simulink model "test_direct"  (R2024a)
settings: Solver=VariableStepAuto  StartTime=0.0  StopTime=40  RelTol=1e-3
libraries: neural x733, simulink x4
(part 12 of 35)

== system test_direct/Function Fitting Neural Network1/Layer 4/Delays 1 ==
  "p{4}" : Inport  PortDimensions=20
      mask Display: e = 0.06;c1 = [120 230 180]/255;c2 = ([120 230 180]+0)/(256+128);c3 = ([120 230 180]+128)/(256+128);patch([0 1 1 0],[0 0 1 1],c1);patch([0 1 1 1-e 1-e 0+e],[0 0 1 1-e 0+e 0+e],c2);patch([0 0 1 1-e 0+e 0+e],[0 1 1 1-e 1-e 0+e],c3);plot([0 1 1 0 0],[0 0 1 1 0]);
  mux : Mux  Inputs=1
      mask Display: e = 0.06;c1 = [120 150 230]/255;c2 = ([120 150 230]+0)/383;c3 = ([120 150 230]+128)/383;patch([0 1 1 0],[0 0 1 1],c1);patch([0 1 1 1-e 1-e 0+e],[0 0 1 1-e 0+e 0+e],c2);patch([0 0 1 1-e 0+e 0+e],[0 1 1 1-e 1-e 0+e],c3);plot([0 1 1 0 0],[0 0 1 1 0]);disp('Mux')
  "pd{4,3}" : Outport
      mask Display: e = 0.06;c1 = [120 230 180]/255;c2 = ([120 230 180]+0)/(256+128);c3 = ([120 230 180]+128)/(256+128);patch([0 1 1 0],[0 0 1 1],c1);patch([0 1 1 1-e 1-e 0+e],[0 0 1 1-e 0+e 0+e],c2);patch([0 0 1 1-e 0+e 0+e],[0 1 1 1-e 1-e 0+e],c3);plot([0 1 1 0 0],[0 0 1 1 0]);
  wires:
  "p{4}"/1 -> mux/1
  mux/1 -> "pd{4,3}"/1

== system test_direct/Function Fitting Neural Network1/Layer 4/LW{4,3} ==
  "ad{4,3}" : Inport  PortDimensions=20
      mask Display: e = 0.06;c1 = [120 230 180]/255;c2 = ([120 230 180]+0)/(256+128);c3 = ([120 230 180]+128)/(256+128);patch([0 1 1 0],[0 0 1 1],c1);patch([0 1 1 1-e 1-e 0+e],[0 0 1 1-e 0+e 0+e],c2);patch([0 0 1 1-e 0+e 0+e],[0 1 1 1-e 1-e 0+e],c3);plot([0 1 1 0 0],[0 0 1 1 0]);
  "IW{4,3}(1,:)'" : Constant  Value=[-0.5538978955091093947515901163569651544094085693359375;0.485168151202809372346536065379041247069835662841796875;-0.5241552760058165727485857132705859839916229248046875;0.393694130681727594289753824341460131108760833740234375;-0.226868820201836685068741417126148007810115814208984375;-0.57887128109770780159948344589793123304843902587890625;-0.0783114975214572461847950535229756496846675872802734375;-0.045766236741898003170803121975040994584560394287109375;0.399668940356752655507222016240120865404605865478515625;0.1856571666806976772523540830661659128963947296142578125;0.10022603350572274749641366042851586826145648956298828125;-0.534264069916555950356951143476180732250213623046875;-0.32018358640142363658043223040294833481311798095703125;0.0185677915168835395987034786458025337196886539459228515625;0.191883392055136547948990255463286302983760833740234375;-0.2105355645822364618613420361725729890167713165283203125;-0.5841688118866372736448511204798705875873565673828125;-0.1594929997566735535574622417698265053331851959228515625;-0.335012858362053245198097783941193483769893646240234375;0.115969582185506958627030371644650585949420928955078125]
      mask Display: e = 0.06;c1 = [120 150 230]/255;c2 = ([120 150 230]+0)/383;c3 = ([120 150 230]+128)/383;patch([0 1 1 0],[0 0 1 1],c1);patch([0 1 1 1-e 1-e 0+e],[0 0 1 1-e 0+e 0+e],c2);patch([0 0 1 1-e 0+e 0+e],[0 1 1 1-e 1-e 0+e],c3);plot([0 1 1 0 0],[0 0 1 1 0]);disp('weights');
  "IW{4,3}(10,:)'" : Constant  Value=[-0.11432279213753747393322868219911470077931880950927734375;-0.482351266656278365729804136208258569240570068359375;-0.401522130496478724115405611883033998310565948486328125;0.240701254689964783128885983387590385973453521728515625;0.463959354447395833087597338817431591451168060302734375;-0.0857875597282283519628975909654400311410427093505859375;-0.464149306377789672151124023002921603620052337646484375;-0.08157369651331071447319942535614245571196079254150390625;-0.0184508443188259076139789982562433579005300998687744140625;0.10195442949925893894036477149711572565138339996337890625;-0.44268411642938565453420096673653461039066314697265625;0.07689143542623187721485322754233493469655513763427734375;-0.5351185554038793146247598997433669865131378173828125;-0.55882335224635160120243426717934198677539825439453125;-0.3511500841433623509857397948508150875568389892578125;0.053339980043120759078956183429909287951886653900146484375;0.250608480405577427330143791550653986632823944091796875;-0.48472883013925793793674756670952774584293365478515625;-0.4930568315285324132446476141922175884246826171875;-0.260318494558593072074614838129491545259952545166015625]
      mask Display: e = 0.06;c1 = [120 150 230]/255;c2 = ([120 150 230]+0)/383;c3 = ([120 150 230]+128)/383;patch([0 1 1 0],[0 0 1 1],c1);patch([0 1 1 1-e 1-e 0+e],[0 0 1 1-e 0+e 0+e],c2);patch([0 0 1 1-e 0+e 0+e],[0 1 1 1-e 1-e 0+e],c3);plot([0 1 1 0 0],[0 0 1 1 0]);disp('weights');
  "IW{4,3}(2,:)'" : Constant  Value=[0.0127625592697413470233414045651443302631378173828125;-0.2491011110049460575144308904782519675791263580322265625;0.274529221095729691892728396851452998816967010498046875;0.0204354876268000480721287459573431988246738910675048828125;0.1585695336445297753957817121772677637636661529541015625;-0.433717579824423993262172416507382877171039581298828125;0.256549476269036180742233455021050758659839630126953125;-0.59634213250017176211059677370940335094928741455078125;0.467939192879395393642738554262905381619930267333984375;-0.5351803245451469681626122110174037516117095947265625;0.306031635985715144698815493029542267322540283203125;0.60240914911445175849991073846467770636081695556640625;-0.272057168040332530978275826782919466495513916015625;-0.11290972902060793237044578063432709313929080963134765625;-0.272119262681239593160142931083100847899913787841796875;0.33969783556142285618761889054439961910247802734375;-0.336592646572185183462266877540969289839267730712890625;-0.0674673853582745675083742753486149013042449951171875;0.02810640498377771356874887942467466928064823150634765625;-0.56221562973156402609475890130852349102497100830078125]
      mask Display: e = 0.06;c1 = [120 150 230]/255;c2 = ([120 150 230]+0)/383;c3 = ([120 150 230]+128)/383;patch([0 1 1 0],[0 0 1 1],c1);patch([0 1 1 1-e 1-e 0+e],[0 0 1 1-e 0+e 0+e],c2);patch([0 0 1 1-e 0+e 0+e],[0 1 1 1-e 1-e 0+e],c3);plot([0 1 1 0 0],[0 0 1 1 0]);disp('weights');
  "IW{4,3}(3,:)'" : Constant  Value=[0.2188595104604072194565134168442455120384693145751953125;-0.61082191094920623708475204693968407809734344482421875;-0.13949203191923309486099924470181576907634735107421875;0.088990754412494210701112251626909710466861724853515625;-0.2483977615196539534547781613582628779113292694091796875;0.64019161482434838728039494526456110179424285888671875;0.055384886144940685681614667146277497522532939910888671875;0.134629674044515368347418871053378097712993621826171875;-0.334046415075910541059300840061041526496410369873046875;-0.31450471701658344603202976941247470676898956298828125;0.468475534970048623772953533261897973716259002685546875;-0.225258262897470029617608133776229806244373321533203125;-0.79555667711204380854184137206175364553928375244140625;-0.08126200166314166695169518561669974587857723236083984375;0.1439878311287706436072397764291963540017604827880859375;-0.2078792366765220001045832987074390985071659088134765625;0.021330185882841364020112706612053443677723407745361328125;0.2476536176992608362379399977726279757916927337646484375;-0.5857412076640569065233421497396193444728851318359375;0.28403214659155440191540265004732646048069000244140625]
      mask Display: e = 0.06;c1 = [120 150 230]/255;c2 = ([120 150 230]+0)/383;c3 = ([120 150 230]+128)/383;patch([0 1 1 0],[0 0 1 1],c1);patch([0 1 1 1-e 1-e 0+e],[0 0 1 1-e 0+e 0+e],c2);patch([0 0 1 1-e 0+e 0+e],[0 1 1 1-e 1-e 0+e],c3);plot([0 1 1 0 0],[0 0 1 1 0]);disp('weights');
  "IW{4,3}(4,:)'" : Constant  Value=[0.2585820940168688242266625820775516331195831298828125;-0.1737609988183630160829551414281013421714305877685546875;-0.477917027781003478370536186048411764204502105712890625;-0.046308943533362734168434826642624102532863616943359375;0.361513420129663420876653390223509632050991058349609375;0.5260368462259947808234983313013799488544464111328125;0.524811065268491194757416451466269791126251220703125;0.2021890196591214217125553886944544501602649688720703125;-0.48351659091220344777184436679817736148834228515625;-0.1812405031101615160427087403149926103651523590087890625;0.483157544390697524239186577688087709248065948486328125;0.47700293418213834950591945016640238463878631591796875;0.062389517060435363549064646804254152812063694000244140625;0.389286015620072756160396920677158050239086151123046875;-0.343054175438237851647471643445896916091442108154296875;-0.51584121186782205814580493097309954464435577392578125;-0.06241903372680314421305780570037313736975193023681640625;-0.1281789351160332601775593275306164287030696868896484375;0.3810151986269849633259809706942178308963775634765625;-0.025934325027326461665655443766809185035526752471923828125]
      mask Display: e = 0.06;c1 = [120 150 230]/255;c2 = ([120 150 230]+0)/383;c3 = ([120 150 230]+128)/383;patch([0 1 1 0],[0 0 1 1],c1);patch([0 1 1 1-e 1-e 0+e],[0 0 1 1-e 0+e 0+e],c2);patch([0 0 1 1-e 0+e 0+e],[0 1 1 1-e 1-e 0+e],c3);plot([0 1 1 0 0],[0 0 1 1 0]);disp('weights');
  "IW{4,3}(5,:)'" : Constant  Value=[-0.4155409087458796779657177467015571892261505126953125;0.0757908169991367286488781473963172174990177154541015625;0.311161200796664927370471787071437574923038482666015625;0.135559405329110094218236781671294011175632476806640625;0.315182748902958886905167901204549707472324371337890625;-0.183457594430218418057876306193065829575061798095703125;-0.257932112663062707014205443556420505046844482421875;0.350534426975030399820099091812153346836566925048828125;-0.46710597951162424745774615075788460671901702880859375;-0.351375929175340162569085578070371411740779876708984375;-0.3741179625289901000684267273754812777042388916015625;0.171501608502107216747134543766151182353496551513671875;0.56741843887494181064568010697257705032825469970703125;-0.432576571812739507638667646460817195475101470947265625;-0.1685319928234139397194013554326375015079975128173828125;-0.0642144342892413677592600151911028660833835601806640625;-0.305922232565454532693394185116630978882312774658203125;-0.6002978670519263371119222938432358205318450927734375;0.307770125551044604339523402813938446342945098876953125;-0.2420667626862628429851298506036982871592044830322265625]
      mask Display: e = 0.06;c1 = [120 150 230]/255;c2 = ([120 150 230]+0)/383;c3 = ([120 150 230]+128)/383;patch([0 1 1 0],[0 0 1 1],c1);patch([0 1 1 1-e 1-e 0+e],[0 0 1 1-e 0+e 0+e],c2);patch([0 0 1 1-e 0+e 0+e],[0 1 1 1-e 1-e 0+e],c3);plot([0 1 1 0 0],[0 0 1 1 0]);disp('weights');
  "IW{4,3}(6,:)'" : Constant  Value=[-0.45235551590633760188353562625707127153873443603515625;0.027443316657496531763005265247556963004171848297119140625;-0.2056081121966515379284601294784806668758392333984375;-0.56361685326390997818890582493622787296772003173828125;0.43814605710889764633719778430531732738018035888671875;0.222411824511333844345273291764897294342517852783203125;-0.045492048109866102534315501770834089256823062896728515625;0.07564035211335683184241673870928934775292873382568359375;-0.269073117924057025884820859573665075004100799560546875;-0.2163415954024009157929953062193817459046840667724609375;0.093430490766664153756693167451885528862476348876953125;0.3983523707029721361294605230796150863170623779296875;0.384680325863053729218421494806534610688686370849609375;-0.005097318314965250916903638511712415493093430995941162109375;-0.327669612705729085266881384086445905268192291259765625;0.01076263086550180957112754498439244343899190425872802734375;-0.27855831684115550661573479374055750668048858642578125;-0.355704598847734754230032194755040109157562255859375;0.39868187274601030178899918610113672912120819091796875;0.277149546995572648722117037323187105357646942138671875]
      mask Display: e = 0.06;c1 = [120 150 230]/255;c2 = ([120 150 230]+0)/383;c3 = ([120 150 230]+128)/383;patch([0 1 1 0],[0 0 1 1],c1);patch([0 1 1 1-e 1-e 0+e],[0 0 1 1-e 0+e 0+e],c2);patch([0 0 1 1-e 0+e 0+e],[0 1 1 1-e 1-e 0+e],c3);plot([0 1 1 0 0],[0 0 1 1 0]);disp('weights');
  "IW{4,3}(7,:)'" : Constant  Value=[-0.39141431944838245282625166510115377604961395263671875;0.144629568712975442590362717965035699307918548583984375;0.448415623333730251065532002030522562563419342041015625;0.07203543440746544568309417400087113492190837860107421875;-0.049350510573182237994416254878160543739795684814453125;0.60201026048241390586923671435215510427951812744140625;0.52080937916731195880259974728687666356563568115234375;0.1825903973983540595771302150751580484211444854736328125;-0.373030512130486158195452617292176000773906707763671875;0.308631840608573571049788597520091570913791656494140625;-0.39096605149584429117481931825750507414340972900390625;-0.0546620178664551648051173060594010166823863983154296875;-0.6224710510971396271173716741031967103481292724609375;-0.57074858282361196071263975682086311280727386474609375;-0.3197072987470479521476818263181485235691070556640625;0.33407318082064418884868928216747008264064788818359375;0.310634083167630026256489372826763428747653961181640625;0.1737175313627656592085912734546582214534282684326171875;0.29918083783679072507055707319523207843303680419921875;0.250744039394872719750395617666072212159633636474609375]
      mask Display: e = 0.06;c1 = [120 150 230]/255;c2 = ([120 150 230]+0)/383;c3 = ([120 150 230]+128)/383;patch([0 1 1 0],[0 0 1 1],c1);patch([0 1 1 1-e 1-e 0+e],[0 0 1 1-e 0+e 0+e],c2);patch([0 0 1 1-e 0+e 0+e],[0 1 1 1-e 1-e 0+e],c3);plot([0 1 1 0 0],[0 0 1 1 0]);disp('weights');
  "IW{4,3}(8,:)'" : Constant  Value=[0.341408820649164390648167000108514912426471710205078125;-0.386313232066315903612263582544983364641666412353515625;-0.11805065794366853548780227356473915278911590576171875;0.410962077337723774572708634877926670014858245849609375;0.018381337048181768667465263433768996037542819976806640625;0.03465676675159745645515840806183405220508575439453125;0.1011843324394486043349417059289407916367053985595703125;0.489059537655913256770645602955482900142669677734375;0.346112051877071669192531544467783533036708831787109375;-0.10491802612202581757028241327134310267865657806396484375;-0.6823458958969526033655483843176625669002532958984375;-0.258128428044318403156154317912296392023563385009765625;0.137093797283970530997976311482489109039306640625;-0.2007511194004691634784620646314579062163829803466796875;-0.397827808858892961740849614216131158173084259033203125;-0.2758776820591306577767909402609802782535552978515625;0.09431593045098592142938542792762746103107929229736328125;-0.1261406751021386385414047026642947457730770111083984375;-0.57205714082915737339618544865516014397144317626953125;0.475472254725631648941686080434010364115238189697265625]
      mask Display: e = 0.06;c1 = [120 150 230]/255;c2 = ([120 150 230]+0)/383;c3 = ([120 150 230]+128)/383;patch([0 1 1 0],[0 0 1 1],c1);patch([0 1 1 1-e 1-e 0+e],[0 0 1 1-e 0+e 0+e],c2);patch([0 0 1 1-e 0+e 0+e],[0 1 1 1-e 1-e 0+e],c3);plot([0 1 1 0 0],[0 0 1 1 0]);disp('weights');
  "IW{4,3}(9,:)'" : Constant  Value=[0.63220657027571502961649230201146565377712249755859375;-0.515869854384149117976221532444469630718231201171875;-0.042750743473010423267854918094599270261824131011962890625;0.04051288556244121707994310099820722825825214385986328125;0.1568319244851359706149906969585572369396686553955078125;-0.11638208636440784682353211110239499248564243316650390625;0.34595843681200744157422377611510455608367919921875;-0.063768168762912302849343859634245745837688446044921875;-0.5681062739616578038948091489146463572978973388671875;0.39724581896035715544712729752063751220703125;-0.36775156254761764973437720982474274933338165283203125;-0.4264153017873775208812503478839062154293060302734375;-0.2194014740512104932879111629517865367233753204345703125;0.253309338102697012562458667161990888416767120361328125;0.0791363151879848902847669478433090262115001678466796875;0.374882768614814343433039312003529630601406097412109375;-0.492042398606798270233042558174929581582546234130859375;0.5008728219296603167975945325451903045177459716796875;-0.362117147538655259619844173357705585658550262451171875;-0.251333360046878839799688876155414618551731109619140625]
      mask Display: e = 0.06;c1 = [120 150 230]/255;c2 = ([120 150 230]+0)/383;c3 = ([120 150 230]+128)/383;patch([0 1 1 0],[0 0 1 1],c1);patch([0 1 1 1-e 1-e 0+e],[0 0 1 1-e 0+e 0+e],c2);patch([0 0 1 1-e 0+e 0+e],[0 1 1 1-e 1-e 0+e],c3);plot([0 1 1 0 0],[0 0 1 1 0]);disp('weights');
  Mux : Mux  Inputs=10
      mask Display: e = 0.06;c1 = [120 150 230]/255;c2 = ([120 150 230]+0)/383;c3 = ([120 150 230]+128)/383;patch([0 1 1 0],[0 0 1 1],c1);patch([0 1 1 1-e 1-e 0+e],[0 0 1 1-e 0+e 0+e],c2);patch([0 0 1 1-e 0+e 0+e],[0 1 1 1-e 1-e 0+e],c3);plot([0 1 1 0 0],[0 0 1 1 0]);disp('Mux');
  dotprod{1..10} (10 alike) : neural/Weight Functions/dotprod
  "lz{4,3}" : Outport
      mask Display: e = 0.06;c1 = [120 230 180]/255;c2 = ([120 230 180]+0)/(256+128);c3 = ([120 230 180]+128)/(256+128);patch([0 1 1 0],[0 0 1 1],c1);patch([0 1 1 1-e 1-e 0+e],[0 0 1 1-e 0+e 0+e],c2);patch([0 0 1 1-e 0+e 0+e],[0 1 1 1-e 1-e 0+e],c3);plot([0 1 1 0 0],[0 0 1 1 0]);
  wires:
  "IW{4,3}(1,:)'"/1 -> dotprod1/1
  "ad{4,3}"/1 -> dotprod1/2, dotprod2/2, dotprod3/2, dotprod4/2, dotprod5/2, dotprod6/2, dotprod7/2, dotprod8/2, dotprod9/2, dotprod10/2
  dotprod1/1 -> Mux/1
  "IW{4,3}(2,:)'"/1 -> dotprod2/1
  dotprod2/1 -> Mux/2
  "IW{4,3}(3,:)'"/1 -> dotprod3/1
  dotprod3/1 -> Mux/3
  "IW{4,3}(4,:)'"/1 -> dotprod4/1
  dotprod4/1 -> Mux/4
  "IW{4,3}(5,:)'"/1 -> dotprod5/1
  dotprod5/1 -> Mux/5
  "IW{4,3}(6,:)'"/1 -> dotprod6/1
  dotprod6/1 -> Mux/6
  "IW{4,3}(7,:)'"/1 -> dotprod7/1
  dotprod7/1 -> Mux/7
  "IW{4,3}(8,:)'"/1 -> dotprod8/1
  dotprod8/1 -> Mux/8
  "IW{4,3}(9,:)'"/1 -> dotprod9/1
  dotprod9/1 -> Mux/9
  "IW{4,3}(10,:)'"/1 -> dotprod10/1
  dotprod10/1 -> Mux/10
  Mux/1 -> "lz{4,3}"/1

== system test_direct/Function Fitting Neural Network1/Layer 5/Delays 1 ==
  "p{5}" : Inport  PortDimensions=10
      mask Display: e = 0.06;c1 = [120 230 180]/255;c2 = ([120 230 180]+0)/(256+128);c3 = ([120 230 180]+128)/(256+128);patch([0 1 1 0],[0 0 1 1],c1);patch([0 1 1 1-e 1-e 0+e],[0 0 1 1-e 0+e 0+e],c2);patch([0 0 1 1-e 0+e 0+e],[0 1 1 1-e 1-e 0+e],c3);plot([0 1 1 0 0],[0 0 1 1 0]);
  mux : Mux  Inputs=1
      mask Display: e = 0.06;c1 = [120 150 230]/255;c2 = ([120 150 230]+0)/383;c3 = ([120 150 230]+128)/383;patch([0 1 1 0],[0 0 1 1],c1);patch([0 1 1 1-e 1-e 0+e],[0 0 1 1-e 0+e 0+e],c2);patch([0 0 1 1-e 0+e 0+e],[0 1 1 1-e 1-e 0+e],c3);plot([0 1 1 0 0],[0 0 1 1 0]);disp('Mux')
  "pd{5,4}" : Outport
      mask Display: e = 0.06;c1 = [120 230 180]/255;c2 = ([120 230 180]+0)/(256+128);c3 = ([120 230 180]+128)/(256+128);patch([0 1 1 0],[0 0 1 1],c1);patch([0 1 1 1-e 1-e 0+e],[0 0 1 1-e 0+e 0+e],c2);patch([0 0 1 1-e 0+e 0+e],[0 1 1 1-e 1-e 0+e],c3);plot([0 1 1 0 0],[0 0 1 1 0]);
  wires:
  "p{5}"/1 -> mux/1
  mux/1 -> "pd{5,4}"/1

== system test_direct/Function Fitting Neural Network1/Layer 5/LW{5,4} ==
  "ad{5,4}" : Inport  PortDimensions=10
      mask Display: e = 0.06;c1 = [120 230 180]/255;c2 = ([120 230 180]+0)/(256+128);c3 = ([120 230 180]+128)/(256+128);patch([0 1 1 0],[0 0 1 1],c1);patch([0 1 1 1-e 1-e 0+e],[0 0 1 1-e 0+e 0+e],c2);patch([0 0 1 1-e 0+e 0+e],[0 1 1 1-e 1-e 0+e],c3);plot([0 1 1 0 0],[0 0 1 1 0]);
  "IW{5,4}(1,:)'" : Constant  Value=[-0.2370525451489846890940071943987277336418628692626953125;0.79420661219177601797269971939385868608951568603515625;0.77425635090139122151953188222250901162624359130859375;-0.61710790036603768715650630838354118168354034423828125;0.81721017405651996678983550737029872834682464599609375;1.0160871028313531727604868137859739363193511962890625;0.07357193640244376331427389459349797107279300689697265625;0.33866971773571918902234756387770175933837890625;-0.5733331291719505617976437861216254532337188720703125;-0.56063235277897405239855288527905941009521484375]
      mask Display: e = 0.06;c1 = [120 150 230]/255;c2 = ([120 150 230]+0)/383;c3 = ([120 150 230]+128)/383;patch([0 1 1 0],[0 0 1 1],c1);patch([0 1 1 1-e 1-e 0+e],[0 0 1 1-e 0+e 0+e],c2);patch([0 0 1 1-e 0+e 0+e],[0 1 1 1-e 1-e 0+e],c3);plot([0 1 1 0 0],[0 0 1 1 0]);disp('weights');
  "IW{5,4}(2,:)'" : Constant  Value=[0.59928291987501480786448837534408085048198699951171875;0.409032854106810617178524580594967119395732879638671875;0.606415191800084851792007611948065459728240966796875;0.52728855882009029176771264246781356632709503173828125;0.563048941480805975601242607808671891689300537109375;-0.52108152610402436177849949672236107289791107177734375;-0.756831948750020355731749077676795423030853271484375;0.943526572267819663153431974933482706546783447265625;0.44638115574993142420368030798272229731082916259765625;0.00185134641803159677615753242463370042969472706317901611328125]
      mask Display: e = 0.06;c1 = [120 150 230]/255;c2 = ([120 150 230]+0)/383;c3 = ([120 150 230]+128)/383;patch([0 1 1 0],[0 0 1 1],c1);patch([0 1 1 1-e 1-e 0+e],[0 0 1 1-e 0+e 0+e],c2);patch([0 0 1 1-e 0+e 0+e],[0 1 1 1-e 1-e 0+e],c3);plot([0 1 1 0 0],[0 0 1 1 0]);disp('weights');
  Mux : Mux  Inputs=2
      mask Display: e = 0.06;c1 = [120 150 230]/255;c2 = ([120 150 230]+0)/383;c3 = ([120 150 230]+128)/383;patch([0 1 1 0],[0 0 1 1],c1);patch([0 1 1 1-e 1-e 0+e],[0 0 1 1-e 0+e 0+e],c2);patch([0 0 1 1-e 0+e 0+e],[0 1 1 1-e 1-e 0+e],c3);plot([0 1 1 0 0],[0 0 1 1 0]);disp('Mux');
  dotprod1 : neural/Weight Functions/dotprod
  dotprod2 : neural/Weight Functions/dotprod
  "lz{5,4}" : Outport
      mask Display: e = 0.06;c1 = [120 230 180]/255;c2 = ([120 230 180]+0)/(256+128);c3 = ([120 230 180]+128)/(256+128);patch([0 1 1 0],[0 0 1 1],c1);patch([0 1 1 1-e 1-e 0+e],[0 0 1 1-e 0+e 0+e],c2);patch([0 0 1 1-e 0+e 0+e],[0 1 1 1-e 1-e 0+e],c3);plot([0 1 1 0 0],[0 0 1 1 0]);
  wires:
  "IW{5,4}(1,:)'"/1 -> dotprod1/1
  "ad{5,4}"/1 -> dotprod1/2, dotprod2/2
  dotprod1/1 -> Mux/1
  "IW{5,4}(2,:)'"/1 -> dotprod2/1
  dotprod2/1 -> Mux/2
  Mux/1 -> "lz{5,4}"/1

== system test_direct/Function Fitting Neural Network2/Layer 1/Delays 1 ==
  "p{1}" : Inport  PortDimensions=8
      mask Display: e = 0.06;c1 = [120 230 180]/255;c2 = ([120 230 180]+0)/(256+128);c3 = ([120 230 180]+128)/(256+128);patch([0 1 1 0],[0 0 1 1],c1);patch([0 1 1 1-e 1-e 0+e],[0 0 1 1-e 0+e 0+e],c2);patch([0 0 1 1-e 0+e 0+e],[0 1 1 1-e 1-e 0+e],c3);plot([0 1 1 0 0],[0 0 1 1 0]);
  mux : Mux  Inputs=1
      mask Display: e = 0.06;c1 = [120 150 230]/255;c2 = ([120 150 230]+0)/383;c3 = ([120 150 230]+128)/383;patch([0 1 1 0],[0 0 1 1],c1);patch([0 1 1 1-e 1-e 0+e],[0 0 1 1-e 0+e 0+e],c2);patch([0 0 1 1-e 0+e 0+e],[0 1 1 1-e 1-e 0+e],c3);plot([0 1 1 0 0],[0 0 1 1 0]);disp('Mux')
  "pd{1,1}" : Outport
      mask Display: e = 0.06;c1 = [120 230 180]/255;c2 = ([120 230 180]+0)/(256+128);c3 = ([120 230 180]+128)/(256+128);patch([0 1 1 0],[0 0 1 1],c1);patch([0 1 1 1-e 1-e 0+e],[0 0 1 1-e 0+e 0+e],c2);patch([0 0 1 1-e 0+e 0+e],[0 1 1 1-e 1-e 0+e],c3);plot([0 1 1 0 0],[0 0 1 1 0]);
  wires:
  "p{1}"/1 -> mux/1
  mux/1 -> "pd{1,1}"/1

== system test_direct/Function Fitting Neural Network2/Layer 1/IW{1,1} ==
  "pd{1,1}" : Inport  PortDimensions=8
      mask Display: e = 0.06;c1 = [120 230 180]/255;c2 = ([120 230 180]+0)/(256+128);c3 = ([120 230 180]+128)/(256+128);patch([0 1 1 0],[0 0 1 1],c1);patch([0 1 1 1-e 1-e 0+e],[0 0 1 1-e 0+e 0+e],c2);patch([0 0 1 1-e 0+e 0+e],[0 1 1 1-e 1-e 0+e],c3);plot([0 1 1 0 0],[0 0 1 1 0]);
  "IW{1,1}(1,:)'" : Constant  Value=[0.7018721038438353598820640399935655295848846435546875;-0.78272020959444288390471911043277941644191741943359375;0.287312516828068631458137360823457129299640655517578125;0.100321628581366006915942534760688431560993194580078125;-0.68574331266115529093241320879315026104450225830078125;1.1061476627284509977044990591821260750293731689453125;-0.53704899534238659253304604135337285697460174560546875;-0.12017958469422394818248989167841500602662563323974609375]
      mask Display: e = 0.06;c1 = [120 150 230]/255;c2 = ([120 150 230]+0)/383;c3 = ([120 150 230]+128)/383;patch([0 1 1 0],[0 0 1 1],c1);patch([0 1 1 1-e 1-e 0+e],[0 0 1 1-e 0+e 0+e],c2);patch([0 0 1 1-e 0+e 0+e],[0 1 1 1-e 1-e 0+e],c3);plot([0 1 1 0 0],[0 0 1 1 0]);disp('Weights');
  "IW{1,1}(10,:)'" : Constant  Value=[0.01004118264387344854060568621889615315012633800506591796875;0.55679567162215992670581954371300525963306427001953125;-0.83175967038832887556765172121231444180011749267578125;-0.2294582581958591604998076718402444384992122650146484375;0.66995366070517847756349283372401259839534759521484375;1.0460062130397764779132785406545735895633697509765625;-0.5889707813277176295940762429381720721721649169921875;-1.1942740236180007240562872539157979190349578857421875]
      mask Display: e = 0.06;c1 = [120 150 230]/255;c2 = ([120 150 230]+0)/383;c3 = ([120 150 230]+128)/383;patch([0 1 1 0],[0 0 1 1],c1);patch([0 1 1 1-e 1-e 0+e],[0 0 1 1-e 0+e 0+e],c2);patch([0 0 1 1-e 0+e 0+e],[0 1 1 1-e 1-e 0+e],c3);plot([0 1 1 0 0],[0 0 1 1 0]);disp('Weights');
  "IW{1,1}(11,:)'" : Constant  Value=[-0.4150065618707252657060280398582108318805694580078125;0.772807290396359203299425644217990338802337646484375;0.7462491824195780498740759867359884083271026611328125;0.5864789456728105587757227112888358533382415771484375;-0.37684577916515216156057022089953534305095672607421875;0.9280146778236206817069842145428992807865142822265625;0.348609392479936719411170997773297131061553955078125;-0.06447739869570746906735081438455381430685520172119140625]
      mask Display: e = 0.06;c1 = [120 150 230]/255;c2 = ([120 150 230]+0)/383;c3 = ([120 150 230]+128)/383;patch([0 1 1 0],[0 0 1 1],c1);patch([0 1 1 1-e 1-e 0+e],[0 0 1 1-e 0+e 0+e],c2);patch([0 0 1 1-e 0+e 0+e],[0 1 1 1-e 1-e 0+e],c3);plot([0 1 1 0 0],[0 0 1 1 0]);disp('Weights');
  "IW{1,1}(12,:)'" : Constant  Value=[0.225553434401855046331775156431831419467926025390625;-0.28382172302285979537117555082659237086772918701171875;-0.45266791120581506557840612003928981721401214599609375;-1.009913788724838834554020650102756917476654052734375;0.3425240274380125793385332144680432975292205810546875;-1.3627690304660216025212093882146291434764862060546875;0.331756255307284975142323446561931632459163665771484375;0.35554188979848355689483696551178582012653350830078125]
      mask Display: e = 0.06;c1 = [120 150 230]/255;c2 = ([120 150 230]+0)/383;c3 = ([120 150 230]+128)/383;patch([0 1 1 0],[0 0 1 1],c1);patch([0 1 1 1-e 1-e 0+e],[0 0 1 1-e 0+e 0+e],c2);patch([0 0 1 1-e 0+e 0+e],[0 1 1 1-e 1-e 0+e],c3);plot([0 1 1 0 0],[0 0 1 1 0]);disp('Weights');
  "IW{1,1}(13,:)'" : Constant  Value=[-0.061326752522184592442133777012713835574686527252197265625;-0.12510530582424994605617030174471437931060791015625;-0.65933590772088213061152828231570310890674591064453125;0.339016681429591237861842500933562405407428741455078125;0.265510826939598765239480826494400389492511749267578125;0.451275026974948756386396553352824412286281585693359375;-0.356608199330063990739603241308941505849361419677734375;1.3974919367716920337585406741709448397159576416015625]
      mask Display: e = 0.06;c1 = [120 150 230]/255;c2 = ([120 150 230]+0)/383;c3 = ([120 150 230]+128)/383;patch([0 1 1 0],[0 0 1 1],c1);patch([0 1 1 1-e 1-e 0+e],[0 0 1 1-e 0+e 0+e],c2);patch([0 0 1 1-e 0+e 0+e],[0 1 1 1-e 1-e 0+e],c3);plot([0 1 1 0 0],[0 0 1 1 0]);disp('Weights');
  "IW{1,1}(14,:)'" : Constant  Value=[-0.0890354198141431740776141623427974991500377655029296875;0.471981245562988871444787264408660121262073516845703125;-0.07579474757898187198268402653411612845957279205322265625;-0.28060834554075364533076708539738319814205169677734375;0.4229168228938904317004698896198533475399017333984375;-0.327695834352655868126902305448311381042003631591796875;-1.306448755615633228188698922167532145977020263671875;1.0364717755299832635529355684411711990833282470703125]
      mask Display: e = 0.06;c1 = [120 150 230]/255;c2 = ([120 150 230]+0)/383;c3 = ([120 150 230]+128)/383;patch([0 1 1 0],[0 0 1 1],c1);patch([0 1 1 1-e 1-e 0+e],[0 0 1 1-e 0+e 0+e],c2);patch([0 0 1 1-e 0+e 0+e],[0 1 1 1-e 1-e 0+e],c3);plot([0 1 1 0 0],[0 0 1 1 0]);disp('Weights');
  "IW{1,1}(15,:)'" : Constant  Value=[-0.430734202476834970862995533025241456925868988037109375;0.347240742961757831164248955246875993907451629638671875;-0.9286241410400484230791562367812730371952056884765625;-0.1538992271100617925672082719756872393190860748291015625;-0.55801758357549580136236500038648955523967742919921875;0.1611475206759109546350572372830356471240520477294921875;-0.8689828741968572689557959165540523827075958251953125;-0.51739154752782778867725710369995795190334320068359375]
      mask Display: e = 0.06;c1 = [120 150 230]/255;c2 = ([120 150 230]+0)/383;c3 = ([120 150 230]+128)/383;patch([0 1 1 0],[0 0 1 1],c1);patch([0 1 1 1-e 1-e 0+e],[0 0 1 1-e 0+e 0+e],c2);patch([0 0 1 1-e 0+e 0+e],[0 1 1 1-e 1-e 0+e],c3);plot([0 1 1 0 0],[0 0 1 1 0]);disp('Weights');
  "IW{1,1}(16,:)'" : Constant  Value=[-0.05770924535914423447735543959424830973148345947265625;1.109060552360722429199313410208560526371002197265625;0.2053137265425397373075355744731496088206768035888671875;0.152573486913419653632217887206934392452239990234375;-0.60614333166010381237498449991107918322086334228515625;1.3568119523186246144774713684455491602420806884765625;-0.022061332740077370384579324991136672906577587127685546875;-0.323243349065083729332314987914287485182285308837890625]
      mask Display: e = 0.06;c1 = [120 150 230]/255;c2 = ([120 150 230]+0)/383;c3 = ([120 150 230]+128)/383;patch([0 1 1 0],[0 0 1 1],c1);patch([0 1 1 1-e 1-e 0+e],[0 0 1 1-e 0+e 0+e],c2);patch([0 0 1 1-e 0+e 0+e],[0 1 1 1-e 1-e 0+e],c3);plot([0 1 1 0 0],[0 0 1 1 0]);disp('Weights');
  "IW{1,1}(17,:)'" : Constant  Value=[-0.0927600123262486142561300539455260150134563446044921875;0.2371070489635958844498730968552990816533565521240234375;-0.448744648118801270353372956378734670579433441162109375;-0.2047515696996531631146609697680105455219745635986328125;0.50108715633369216302384074879228137433528900146484375;1.1857982110989351287599902207148261368274688720703125;0.84320171558148693247147775764460675418376922607421875;-1.135275279571598350258909704280085861682891845703125]
      mask Display: e = 0.06;c1 = [120 150 230]/255;c2 = ([120 150 230]+0)/383;c3 = ([120 150 230]+128)/383;patch([0 1 1 0],[0 0 1 1],c1);patch([0 1 1 1-e 1-e 0+e],[0 0 1 1-e 0+e 0+e],c2);patch([0 0 1 1-e 0+e 0+e],[0 1 1 1-e 1-e 0+e],c3);plot([0 1 1 0 0],[0 0 1 1 0]);disp('Weights');
  "IW{1,1}(18,:)'" : Constant  Value=[-0.1014621720080778610739713485600077547132968902587890625;0.2615862202668306490949134968104772269725799560546875;0.50917060427266591648987059670616872608661651611328125;0.96994592076268781877246283329441212117671966552734375;1.129229567515210863604124824632890522480010986328125;0.93363361641153375103385769762098789215087890625;0.63886475409989074147887322396854870021343231201171875;0.323744732930749290478189550412935204803943634033203125]
      mask Display: e = 0.06;c1 = [120 150 230]/255;c2 = ([120 150 230]+0)/383;c3 = ([120 150 230]+128)/383;patch([0 1 1 0],[0 0 1 1],c1);patch([0 1 1 1-e 1-e 0+e],[0 0 1 1-e 0+e 0+e],c2);patch([0 0 1 1-e 0+e 0+e],[0 1 1 1-e 1-e 0+e],c3);plot([0 1 1 0 0],[0 0 1 1 0]);disp('Weights');
  "IW{1,1}(19,:)'" : Constant  Value=[0.6414270757818278934081490660901181399822235107421875;-0.299744354329730011698984526447020471096038818359375;-0.75276876511161605609601110700168646872043609619140625;-0.17013525028104059533262670811382122337818145751953125;-0.49154643232037986688709452209877781569957733154296875;-0.34198450101213928586929569064523093402385711669921875;1.2268466059027824943683526726090349256992340087890625;-0.70385621658948116508014436476514674723148345947265625]
      mask Display: e = 0.06;c1 = [120 150 230]/255;c2 = ([120 150 230]+0)/383;c3 = ([120 150 230]+128)/383;patch([0 1 1 0],[0 0 1 1],c1);patch([0 1 1 1-e 1-e 0+e],[0 0 1 1-e 0+e 0+e],c2);patch([0 0 1 1-e 0+e 0+e],[0 1 1 1-e 1-e 0+e],c3);plot([0 1 1 0 0],[0 0 1 1 0]);disp('Weights');
  "IW{1,1}(2,:)'" : Constant  Value=[0.431589302123029039393031780491583049297332763671875;-0.6067521413782841488426811338285915553569793701171875;0.61456729391360920278231105839950032532215118408203125;-0.92312861849797001045914157657534815371036529541015625;-0.880998102223056189785665992530994117259979248046875;0.51885851064652033226565208678948692977428436279296875;-0.50519046378317689072190432852949015796184539794921875;-0.65541986610833358195549180891248397529125213623046875]
      mask Display: e = 0.06;c1 = [120 150 230]/255;c2 = ([120 150 230]+0)/383;c3 = ([120 150 230]+128)/383;patch([0 1 1 0],[0 0 1 1],c1);patch([0 1 1 1-e 1-e 0+e],[0 0 1 1-e 0+e 0+e],c2);patch([0 0 1 1-e 0+e 0+e],[0 1 1 1-e 1-e 0+e],c3);plot([0 1 1 0 0],[0 0 1 1 0]);disp('Weights');
  "IW{1,1}(20,:)'" : Constant  Value=[0.3495156441232165622778893521171994507312774658203125;-0.483608607045198424234655476539046503603458404541015625;-0.073974751010546402341105931554920971393585205078125;-0.465370660978524697259928188941557891666889190673828125;0.9547266235844016346590024113538675010204315185546875;-0.4676375759594904035765239314059726893901824951171875;0.73834359997694554156311141923652030527591705322265625;1.07688416584620672011851638671942055225372314453125]
      mask Display: e = 0.06;c1 = [120 150 230]/255;c2 = ([120 150 230]+0)/383;c3 = ([120 150 230]+128)/383;patch([0 1 1 0],[0 0 1 1],c1);patch([0 1 1 1-e 1-e 0+e],[0 0 1 1-e 0+e 0+e],c2);patch([0 0 1 1-e 0+e 0+e],[0 1 1 1-e 1-e 0+e],c3);plot([0 1 1 0 0],[0 0 1 1 0]);disp('Weights');
  "IW{1,1}(3,:)'" : Constant  Value=[-0.1319230513033761986729786030991817824542522430419921875;0.6795771293588248607164814529824070632457733154296875;0.56343328067635767286702730416436679661273956298828125;0.00704642403237338253718657909985267906449735164642333984375;1.0174831437031188752229127203463576734066009521484375;0.83056998366831802371734738699160516262054443359375;0.186372878266695740645531031987047754228115081787109375;-1.2091872158942791326552423925022594630718231201171875]
      mask Display: e = 0.06;c1 = [120 150 230]/255;c2 = ([120 150 230]+0)/383;c3 = ([120 150 230]+128)/383;patch([0 1 1 0],[0 0 1 1],c1);patch([0 1 1 1-e 1-e 0+e],[0 0 1 1-e 0+e 0+e],c2);patch([0 0 1 1-e 0+e 0+e],[0 1 1 1-e 1-e 0+e],c3);plot([0 1 1 0 0],[0 0 1 1 0]);disp('Weights');
  "IW{1,1}(4,:)'" : Constant  Value=[0.282335772428924658417059845305630005896091461181640625;0.1573612105347056699944374713595607317984104156494140625;-1.0364364516919122305438349940232001245021820068359375;0.662730391421358699943766623619012534618377685546875;0.56457167291433585365467706651543267071247100830078125;-0.8382631797901769488134959829039871692657470703125;-0.700147569233711575265033388859592378139495849609375;0.406430481243703456417648567366995848715305328369140625]
      mask Display: e = 0.06;c1 = [120 150 230]/255;c2 = ([120 150 230]+0)/383;c3 = ([120 150 230]+128)/383;patch([0 1 1 0],[0 0 1 1],c1);patch([0 1 1 1-e 1-e 0+e],[0 0 1 1-e 0+e 0+e],c2);patch([0 0 1 1-e 0+e 0+e],[0 1 1 1-e 1-e 0+e],c3);plot([0 1 1 0 0],[0 0 1 1 0]);disp('Weights');
  "IW{1,1}(5,:)'" : Constant  Value=[0.351759382210662663315048348522395826876163482666015625;-0.2163994278951308636305128629828686825931072235107421875;-0.93024073444000965338318565045483410358428955078125;-0.70992317455837916639893592218868434429168701171875;0.2250948504528511862066153526029665954411029815673828125;0.81518825003912265270145098838838748633861541748046875;0.8946882115561114456880886791623197495937347412109375;-0.8939438090499927103138588790898211300373077392578125]
      mask Display: e = 0.06;c1 = [120 150 230]/255;c2 = ([120 150 230]+0)/383;c3 = ([120 150 230]+128)/383;patch([0 1 1 0],[0 0 1 1],c1);patch([0 1 1 1-e 1-e 0+e],[0 0 1 1-e 0+e 0+e],c2);patch([0 0 1 1-e 0+e 0+e],[0 1 1 1-e 1-e 0+e],c3);plot([0 1 1 0 0],[0 0 1 1 0]);disp('Weights');
  "IW{1,1}(6,:)'" : Constant  Value=[-0.0109644393345748013268714515788815333507955074310302734375;-0.846023268464537014921234003850258886814117431640625;0.34354583673125971277073631426901556551456451416015625;0.5337262416938621800710507159237749874591827392578125;0.254651499787102053584675331876496784389019012451171875;0.8717335800958394553816788175026886165142059326171875;0.43224771404483697256893037774716503918170928955078125;-1.2179013816384713919660498504526913166046142578125]
      mask Display: e = 0.06;c1 = [120 150 230]/255;c2 = ([120 150 230]+0)/383;c3 = ([120 150 230]+128)/383;patch([0 1 1 0],[0 0 1 1],c1);patch([0 1 1 1-e 1-e 0+e],[0 0 1 1-e 0+e 0+e],c2);patch([0 0 1 1-e 0+e 0+e],[0 1 1 1-e 1-e 0+e],c3);plot([0 1 1 0 0],[0 0 1 1 0]);disp('Weights');
  "IW{1,1}(7,:)'" : Constant  Value=[-0.9210953153003165194689927375293336808681488037109375;-0.0311384589704766616413689206410708720795810222625732421875;0.038830582294343378435552693872523377649486064910888671875;0.623381048177447549818452898762188851833343505859375;0.16957428934719820379228849560604430735111236572265625;0.79683355714869719133019998480449430644512176513671875;0.790574896457508113911671898677013814449310302734375;0.67705549863605585247938734028139151632785797119140625]
      mask Display: e = 0.06;c1 = [120 150 230]/255;c2 = ([120 150 230]+0)/383;c3 = ([120 150 230]+128)/383;patch([0 1 1 0],[0 0 1 1],c1);patch([0 1 1 1-e 1-e 0+e],[0 0 1 1-e 0+e 0+e],c2);patch([0 0 1 1-e 0+e 0+e],[0 1 1 1-e 1-e 0+e],c3);plot([0 1 1 0 0],[0 0 1 1 0]);disp('Weights');
  "IW{1,1}(8,:)'" : Constant  Value=[-0.2350570428730714145348912325061974115669727325439453125;-0.0308513801393720359100836247989718685857951641082763671875;-0.435990115964150104499452709205797873437404632568359375;0.056236684380723107878896627198628266341984272003173828125;-0.821557828044752636031944348360411822795867919921875;1.2855637677084004177885390163282863795757293701171875;-1.269565743323525008889873788575641810894012451171875;0.06370591353200623363495225248698261566460132598876953125]
      mask Display: e = 0.06;c1 = [120 150 230]/255;c2 = ([120 150 230]+0)/383;c3 = ([120 150 230]+128)/383;patch([0 1 1 0],[0 0 1 1],c1);patch([0 1 1 1-e 1-e 0+e],[0 0 1 1-e 0+e 0+e],c2);patch([0 0 1 1-e 0+e 0+e],[0 1 1 1-e 1-e 0+e],c3);plot([0 1 1 0 0],[0 0 1 1 0]);disp('Weights');
  "IW{1,1}(9,:)'" : Constant  Value=[-0.10740998250970346106214492465369403362274169921875;-0.08402128342254171211589408585496130399405956268310546875;-0.487026686311012479979609679503482766449451446533203125;-0.98840754619886073140122562108444981276988983154296875;-0.9861755278853312489673044183291494846343994140625;-0.219819184952295076929118522457429207861423492431640625;-1.0417457281164050897359629743732511997222900390625;0.6995996561861070883736601899727247655391693115234375]
      mask Display: e = 0.06;c1 = [120 150 230]/255;c2 = ([120 150 230]+0)/383;c3 = ([120 150 230]+128)/383;patch([0 1 1 0],[0 0 1 1],c1);patch([0 1 1 1-e 1-e 0+e],[0 0 1 1-e 0+e 0+e],c2);patch([0 0 1 1-e 0+e 0+e],[0 1 1 1-e 1-e 0+e],c3);plot([0 1 1 0 0],[0 0 1 1 0]);disp('Weights');
  Mux : Mux  Inputs=20
      mask Display: e = 0.06;c1 = [120 150 230]/255;c2 = ([120 150 230]+0)/383;c3 = ([120 150 230]+128)/383;patch([0 1 1 0],[0 0 1 1],c1);patch([0 1 1 1-e 1-e 0+e],[0 0 1 1-e 0+e 0+e],c2);patch([0 0 1 1-e 0+e 0+e],[0 1 1 1-e 1-e 0+e],c3);plot([0 1 1 0 0],[0 0 1 1 0]);disp('Mux');
  dotprod{1..20} (20 alike) : neural/Weight Functions/dotprod
  "iz{1,1}" : Outport
      mask Display: e = 0.06;c1 = [120 230 180]/255;c2 = ([120 230 180]+0)/(256+128);c3 = ([120 230 180]+128)/(256+128);patch([0 1 1 0],[0 0 1 1],c1);patch([0 1 1 1-e 1-e 0+e],[0 0 1 1-e 0+e 0+e],c2);patch([0 0 1 1-e 0+e 0+e],[0 1 1 1-e 1-e 0+e],c3);plot([0 1 1 0 0],[0 0 1 1 0]);
  wires:
  "IW{1,1}(1,:)'"/1 -> dotprod1/1
  "pd{1,1}"/1 -> dotprod1/2, dotprod2/2, dotprod3/2, dotprod4/2, dotprod5/2, dotprod6/2, dotprod7/2, dotprod8/2, dotprod9/2, dotprod10/2, dotprod11/2, dotprod12/2, dotprod13/2, dotprod14/2, dotprod15/2, dotprod16/2, dotprod17/2, dotprod18/2, dotprod19/2, dotprod20/2
  dotprod1/1 -> Mux/1
  "IW{1,1}(2,:)'"/1 -> dotprod2/1
  dotprod2/1 -> Mux/2
  "IW{1,1}(3,:)'"/1 -> dotprod3/1
  dotprod3/1 -> Mux/3
  "IW{1,1}(4,:)'"/1 -> dotprod4/1
  dotprod4/1 -> Mux/4
  "IW{1,1}(5,:)'"/1 -> dotprod5/1
  dotprod5/1 -> Mux/5
  "IW{1,1}(6,:)'"/1 -> dotprod6/1
  dotprod6/1 -> Mux/6
  "IW{1,1}(7,:)'"/1 -> dotprod7/1
  dotprod7/1 -> Mux/7
  "IW{1,1}(8,:)'"/1 -> dotprod8/1
  dotprod8/1 -> Mux/8
  "IW{1,1}(9,:)'"/1 -> dotprod9/1
  dotprod9/1 -> Mux/9
  "IW{1,1}(10,:)'"/1 -> dotprod10/1
  dotprod10/1 -> Mux/10
  "IW{1,1}(11,:)'"/1 -> dotprod11/1
  dotprod11/1 -> Mux/11
  "IW{1,1}(12,:)'"/1 -> dotprod12/1
  dotprod12/1 -> Mux/12
  "IW{1,1}(13,:)'"/1 -> dotprod13/1
  dotprod13/1 -> Mux/13
  "IW{1,1}(14,:)'"/1 -> dotprod14/1
  dotprod14/1 -> Mux/14
  "IW{1,1}(15,:)'"/1 -> dotprod15/1
  dotprod15/1 -> Mux/15
  "IW{1,1}(16,:)'"/1 -> dotprod16/1
  dotprod16/1 -> Mux/16
  "IW{1,1}(17,:)'"/1 -> dotprod17/1
  dotprod17/1 -> Mux/17
  "IW{1,1}(18,:)'"/1 -> dotprod18/1
  dotprod18/1 -> Mux/18
  "IW{1,1}(19,:)'"/1 -> dotprod19/1
  dotprod19/1 -> Mux/19
  "IW{1,1}(20,:)'"/1 -> dotprod20/1
  dotprod20/1 -> Mux/20
  Mux/1 -> "iz{1,1}"/1

== system test_direct/Function Fitting Neural Network2/Layer 2/Delays 1 ==
  "p{2}" : Inport  PortDimensions=20
      mask Display: e = 0.06;c1 = [120 230 180]/255;c2 = ([120 230 180]+0)/(256+128);c3 = ([120 230 180]+128)/(256+128);patch([0 1 1 0],[0 0 1 1],c1);patch([0 1 1 1-e 1-e 0+e],[0 0 1 1-e 0+e 0+e],c2);patch([0 0 1 1-e 0+e 0+e],[0 1 1 1-e 1-e 0+e],c3);plot([0 1 1 0 0],[0 0 1 1 0]);
  mux : Mux  Inputs=1
      mask Display: e = 0.06;c1 = [120 150 230]/255;c2 = ([120 150 230]+0)/383;c3 = ([120 150 230]+128)/383;patch([0 1 1 0],[0 0 1 1],c1);patch([0 1 1 1-e 1-e 0+e],[0 0 1 1-e 0+e 0+e],c2);patch([0 0 1 1-e 0+e 0+e],[0 1 1 1-e 1-e 0+e],c3);plot([0 1 1 0 0],[0 0 1 1 0]);disp('Mux')
  "pd{2,1}" : Outport
      mask Display: e = 0.06;c1 = [120 230 180]/255;c2 = ([120 230 180]+0)/(256+128);c3 = ([120 230 180]+128)/(256+128);patch([0 1 1 0],[0 0 1 1],c1);patch([0 1 1 1-e 1-e 0+e],[0 0 1 1-e 0+e 0+e],c2);patch([0 0 1 1-e 0+e 0+e],[0 1 1 1-e 1-e 0+e],c3);plot([0 1 1 0 0],[0 0 1 1 0]);
  wires:
  "p{2}"/1 -> mux/1
  mux/1 -> "pd{2,1}"/1
